simulink model "geostationary_satellite_ctrl"  (R2020a)
settings: Solver=daessc  StartTime=0.0  StopTime=simlength  MaxStep=ts  RelTol=1e-3
values from neighbouring files (symbols this model uses):
  A = [0 1 0 0; 3*omega_0^2 0 0 2*vt; 0 0 0 1; 0 -2*omega_0/r0 0 0]    [init_satellite_ctrl.m]
  B = 1/ms*[0 0; 1 0; 0 0; 0 1/r0]    [init_satellite_ctrl.m]
  C = [1 0 0 0; 0 0 1 0]    [init_satellite_ctrl.m]
  L = (place(A',C',poles)*19)'    [init_satellite_ctrl.m]
  omega_0 = 7.291e-5    (= 7.291e-05)    [init_satellite_ctrl.m]
  r0 = 4.22e7    (= 42200000)    [init_satellite_ctrl.m]
libraries: nesl_utility x5, geostationary_satellite_lib x1
settings Model: Creator=dbagn  LastModifiedBy=dbagn
settings DataIOCC: ReturnWorkspaceOutputs=off

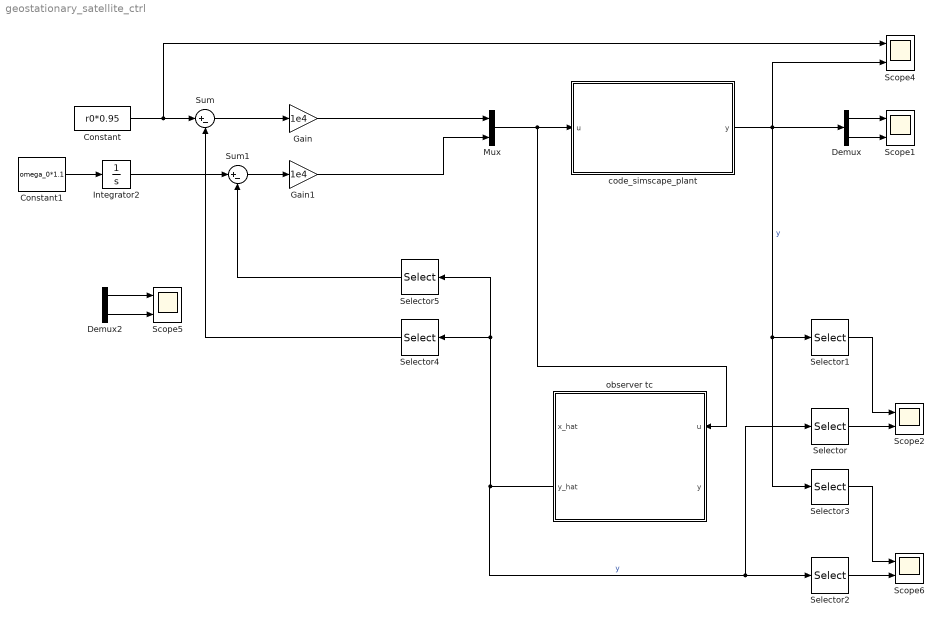
== system geostationary_satellite_ctrl ==
  Constant : Constant  Value=r0*0.95
  Constant1 : Constant  Value=omega_0*1.1
  Demux : Demux  Outputs=2
  Demux2 : Demux  Outputs=2
  Gain : Gain  Gain=1e4
  Gain1 : Gain  Gain=1e4
  Integrator2 : Integrator
  Mux : Mux  Inputs=2
  Scope{1..2,4..6} (5 alike) : Scope  NumInputPorts=2
  Selector : Selector  InputPortWidth=2  IndexOptions=Index vector (dialog)  Indices=1  OutputSizes=1
  Selector1 : Selector  InputPortWidth=2  IndexOptions=Index vector (dialog)  Indices=1  OutputSizes=1
  Selector2 : Selector  InputPortWidth=2  IndexOptions=Index vector (dialog)  Indices=2  OutputSizes=1
  Selector3 : Selector  InputPortWidth=2  IndexOptions=Index vector (dialog)  Indices=2  OutputSizes=1
  Selector4 : Selector  InputPortWidth=2  IndexOptions=Index vector (dialog)  Indices=1  OutputSizes=1
  Selector5 : Selector  InputPortWidth=2  IndexOptions=Index vector (dialog)  Indices=2  OutputSizes=1
  Sum : Sum  Inputs=|+-
  Sum1 : Sum  Inputs=|+-
  "code_simscape_plant " : Subsystem
  observer tc : Subsystem
  wires:
  "code_simscape_plant "/1(y) -> Selector3/1, Selector1/1, Scope4/2, Demux/1  "y"
  Constant1/1 -> Integrator2/1
  Demux/1 -> Scope1/1
  Demux/2 -> Scope1/2
  Selector/1 -> Scope2/2
  Selector1/1 -> Scope2/1
  Selector3/1 -> Scope6/1
  Selector2/1 -> Scope6/2
  Demux2/1 -> Scope5/1
  Demux2/2 -> Scope5/2
  Constant/1 -> Sum/1, Scope4/1
  Sum/1 -> Gain/1
  Gain/1 -> Mux/1
  Mux/1 -> observer tc/1(u), "code_simscape_plant "/1(u)
  Integrator2/1 -> Sum1/1
  Selector5/1 -> Sum1/2
  Sum1/1 -> Gain1/1
  Gain1/1 -> Mux/2
  Selector4/1 -> Sum/2
  observer tc/2(y_hat) -> Selector5/1, Selector4/1, Selector2/1, Selector/1  "y"

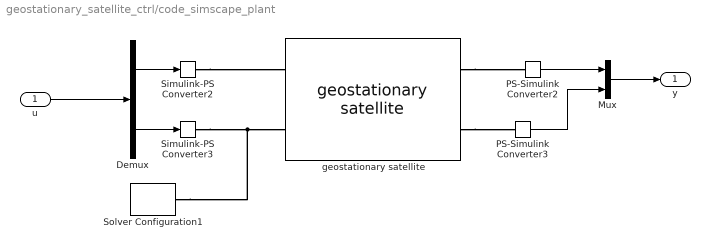
== system geostationary_satellite_ctrl/code_simscape_plant  ==
  u : Inport
  Demux : Demux  Outputs=2
  Mux : Mux  Inputs=2
  PS-Simulink Converter2 : nesl_utility/PS-Simulink Converter  PhysicalDomain=network_engine_domain  SubClassName=ps_output  LeftPortType=input  RightPortType=output  PseudoPeriodic=off  Frequencies=[]  Unit=m  AffineConversion=off
  PS-Simulink Converter3 : nesl_utility/PS-Simulink Converter  PhysicalDomain=network_engine_domain  SubClassName=ps_output  LeftPortType=input  RightPortType=output  PseudoPeriodic=off  Frequencies=[]  Unit=rad  AffineConversion=off
  Simulink-PS Converter2 : nesl_utility/Simulink-PS Converter  PhysicalDomain=network_engine_domain  SubClassName=ps_input  LeftPortType=input  RightPortType=output  PseudoPeriodic=off  Frequencies=[]  NoiseDistribution=none  NoiseParameters=[]  Unit=N  AffineConversion=off  FilteringAndDerivatives=provide  SimscapeFilterOrder=1  InputFilterTimeConstant=0.001  UdotUserProvided=0
  Simulink-PS Converter3 : nesl_utility/Simulink-PS Converter  PhysicalDomain=network_engine_domain  SubClassName=ps_input  LeftPortType=input  RightPortType=output  PseudoPeriodic=off  Frequencies=[]  NoiseDistribution=none  NoiseParameters=[]  Unit=N  AffineConversion=off  FilteringAndDerivatives=provide  SimscapeFilterOrder=1  InputFilterTimeConstant=0.001  UdotUserProvided=0
  Solver Configuration1 : nesl_utility/Solver Configuration  PhysicalDomain=network_engine_domain  SubClassName=solver  LeftPortType=input  RightPortType=generic  Tones=[]  Harmonics=[]  SimulateNoise=off  Profile=off  UseLocalSampling=off  EnableSwitchedLinearOptims=on  FrequencyDomain=off  UseCCode=off  RelTol=0.001  AbsTol=1e-06  MinStep=1e-09  ToWorkspace=off  RevertToSquareIcSolve=off  NumHomotopyIterations=100  PhasorMode=off  PhasorModeNumHarmonics=1  DoDC=off  ResidualTolerance=1e-09  UseLocalSolver=off  LocalSolverChoice=NE_BACKWARD_EULER_ADVANCER  LocalSolverSampleTime=ts  DoFixedCost=off  MaxNonlinIter=3  MaxModeIter=2  LinearAlgebra=auto  EquationFormulation=NE_TIME_EF  DelaysMemoryBudget=1024  AutomaticFiltering=on  FilteringTimeConstant=0.001  PartitionStorageMethod=AS_NEEDED  PartitionMemoryBudget=1024  PartitionMethod=ROBUST
  geostationary satellite : geostationary_satellite_lib/geostationary satellite  Ge=6.673e-11 m^3/kg/s^2  Me=5.97410e24 kg  ms=250 kg  x1_specify=on  x1_priority=High  x1=4.22e+7 m  x1_nominal_specify=off  x1_nominal_unit=m  x1_nominal_value=1  x2_specify=off  x2_priority=None  x2=0 m/s  x2_nominal_specify=off  x2_nominal_unit=m/s  x2_nominal_value=1  x3_specify=off  x3_priority=None  x3=0 rad  x3_nominal_specify=off  x3_nominal_unit=rad  x3_nominal_value=1  x4_specify=on  x4_priority=High  x4=7.291e-5 rad/s  x4_nominal_specify=off  x4_nominal_unit=rad/s  x4_nominal_value=1
      settings: InternalSimscapePortConfiguration="{\"Bottom\":[],\"Left\":[{\"id\":\"ur\",\"label\":\"ur\",\"type\":\"input\"},{\"id\":\"uphi\",\"label\":\"uphi\",\"type\":\"input\"}],\"Right\":[{\"id\":\"r_out\",\"label\":\"r\",\"type\":\"output\"},{\"id\":\"phi_out\",\"label\":\"phi\",\"type\":\"output\"}],\"Top\":[]}"
  y : Outport
  wires:
  Demux/1 -> Simulink-PS Converter2/1
  u/1 -> Demux/1
  Demux/2 -> Simulink-PS Converter3/1
  PS-Simulink Converter2/1 -> Mux/1
  PS-Simulink Converter3/1 -> Mux/2
  Mux/1 -> y/1
  connections:
  Simulink-PS Converter2/RConn1 -- geostationary satellite/LConn1
  Simulink-PS Converter3/RConn1 -- Solver Configuration1/RConn1 -- geostationary satellite/LConn2
  geostationary satellite/RConn1 -- PS-Simulink Converter2/LConn1
  geostationary satellite/RConn2 -- PS-Simulink Converter3/LConn1

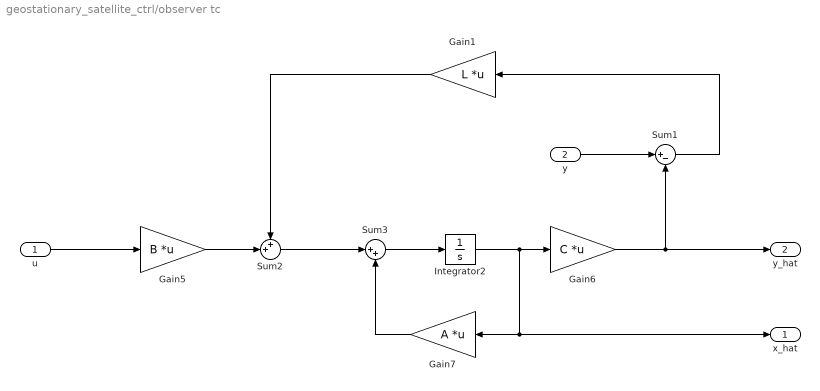
== system geostationary_satellite_ctrl/observer tc ==
  u : Inport
  y : Inport  Port=2
  Gain1 : Gain  Gain=L  Multiplication=Matrix(K*u)
  Gain5 : Gain  Gain=B  Multiplication=Matrix(K*u)
  Gain6 : Gain  Gain=C  Multiplication=Matrix(K*u)
  Gain7 : Gain  Gain=A  Multiplication=Matrix(K*u)
  Integrator2 : Integrator  InitialCondition=[r0 0 0 omega_0]'
  Sum1 : Sum  Inputs=|+-
  Sum2 : Sum  Inputs=++|
  Sum3 : Sum  Inputs=|++
  x_hat : Outport
  y_hat : Outport  Port=2
  wires:
  Sum2/1 -> Sum3/1
  Integrator2/1 -> x_hat/1, Gain7/1, Gain6/1
  Sum3/1 -> Integrator2/1
  Gain7/1 -> Sum3/2
  y/1 -> Sum1/1
  Gain6/1 -> y_hat/1, Sum1/2
  Sum1/1 -> Gain1/1
  u/1 -> Gain5/1
  Gain1/1 -> Sum2/1
  Gain5/1 -> Sum2/2
